simulink model "P702_NI_SoftECU"  (R2019a)
settings: Solver=ode1  StartTime=0.0  StopTime=Inf  FixedStep=0.001  RelTol=1e-3  EnableMultiTasking=on
PreLoadFcn:
  | run '.\VeriStand_BlockSet\NIVeriStandAddPaths.m'
undefined symbols (not defined in the file or in its folder): magnitude
libraries: simulink x83, simulink_extras x1
(part 43 of 76)

== system P702_NI_SoftECU/Input/GWM-SCCM//PDB//RCM//GSM/GSM/Gear_Shift_by_Wire_FD1 ==
  BrkSwtchPos_B_ActlGsm : S-Function  Priority=1  FunctionName=NIVeriStandIO  Parameters=width dtype portnum stime stype btype  SFunctionDeploymentMode=off  EnableBusSupport=off  mask(NI VeriStand Inport){portnum=1, width=-1, stime=-1, dtype=auto, stype=auto, btype=1}
      mask prompts: portnum "Port number:"; width "Port dimensions (-1 for dynamically sized):"; stime "Sample time (-1 for inherited):"; dtype "Data type:"; stype "Signal type:"; btype "Block type:"
      mask help: Use this inport on any level of nested subsystems to allow NI VeriStand software to map signals to it.
      mask init:
      | NIVeriStandIO_init;
      settings: CopyFcn=NIVeriStand_MDL_functions('', 'IO_copy');  DeleteFcn=NIVeriStand_MDL_functions('', 'IO_delete');  MoveFcn=set_param(gcb, 'Mask', 'on');
      mask Callback portnum: NIVeriStand_MDL_functions('', 'IO_setportnum');
      mask TypeOptions dtype: auto | double | single | int8 | uint8 | int16 | uint16 | int32 | uint32 | boolean
      mask Callback dtype: NIVeriStand_MDL_functions('', 'IO_booleansignal');
      mask TypeOptions stype: auto | real | complex
      mask Display:
      | patch([-x x], [-y y], [.90980 .81960 .32156]);
      | plot([xrad -x x xrad], [yrad -y y yrad]);
      | fprintf('NI In%d', portnum);
  Bus_Sig : BusCreator  Inputs=28
  DrQltyDrv_D_StatGsm : S-Function  Priority=2  FunctionName=NIVeriStandIO  Parameters=width dtype portnum stime stype btype  SFunctionDeploymentMode=off  EnableBusSupport=off  mask(NI VeriStand Inport){portnum=2, width=-1, stime=-1, dtype=auto, stype=auto, btype=1}
      mask prompts: portnum "Port number:"; width "Port dimensions (-1 for dynamically sized):"; stime "Sample time (-1 for inherited):"; dtype "Data type:"; stype "Signal type:"; btype "Block type:"
      mask help: Use this inport on any level of nested subsystems to allow NI VeriStand software to map signals to it.
      mask init:
      | NIVeriStandIO_init;
      settings: CopyFcn=NIVeriStand_MDL_functions('', 'IO_copy');  DeleteFcn=NIVeriStand_MDL_functions('', 'IO_delete');  MoveFcn=set_param(gcb, 'Mask', 'on');
      mask Callback portnum: NIVeriStand_MDL_functions('', 'IO_setportnum');
      mask TypeOptions dtype: auto | double | single | int8 | uint8 | int16 | uint16 | int32 | uint32 | boolean
      mask Callback dtype: NIVeriStand_MDL_functions('', 'IO_booleansignal');
      mask TypeOptions stype: auto | real | complex
      mask Display:
      | patch([-x x], [-y y], [.90980 .81960 .32156]);
      | plot([xrad -x x xrad], [yrad -y y yrad]);
      | fprintf('NI In%d', portnum);
  GsmGearMsgTxt_D_Rq : S-Function  Priority=3  FunctionName=NIVeriStandIO  Parameters=width dtype portnum stime stype btype  SFunctionDeploymentMode=off  EnableBusSupport=off  mask(NI VeriStand Inport){portnum=3, width=-1, stime=-1, dtype=auto, stype=auto, btype=1}
      mask prompts: portnum "Port number:"; width "Port dimensions (-1 for dynamically sized):"; stime "Sample time (-1 for inherited):"; dtype "Data type:"; stype "Signal type:"; btype "Block type:"
      mask help: Use this inport on any level of nested subsystems to allow NI VeriStand software to map signals to it.
      mask init:
      | NIVeriStandIO_init;
      settings: CopyFcn=NIVeriStand_MDL_functions('', 'IO_copy');  DeleteFcn=NIVeriStand_MDL_functions('', 'IO_delete');  MoveFcn=set_param(gcb, 'Mask', 'on');
      mask Callback portnum: NIVeriStand_MDL_functions('', 'IO_setportnum');
      mask TypeOptions dtype: auto | double | single | int8 | uint8 | int16 | uint16 | int32 | uint32 | boolean
      mask Callback dtype: NIVeriStand_MDL_functions('', 'IO_booleansignal');
      mask TypeOptions stype: auto | real | complex
      mask Display:
      | patch([-x x], [-y y], [.90980 .81960 .32156]);
      | plot([xrad -x x xrad], [yrad -y y yrad]);
      | fprintf('NI In%d', portnum);
  PrkBrkActv_D_RqGsmGear : S-Function  Priority=4  FunctionName=NIVeriStandIO  Parameters=width dtype portnum stime stype btype  SFunctionDeploymentMode=off  EnableBusSupport=off  mask(NI VeriStand Inport){portnum=4, width=-1, stime=-1, dtype=auto, stype=auto, btype=1}
      mask prompts: portnum "Port number:"; width "Port dimensions (-1 for dynamically sized):"; stime "Sample time (-1 for inherited):"; dtype "Data type:"; stype "Signal type:"; btype "Block type:"
      mask help: Use this inport on any level of nested subsystems to allow NI VeriStand software to map signals to it.
      mask init:
      | NIVeriStandIO_init;
      settings: CopyFcn=NIVeriStand_MDL_functions('', 'IO_copy');  DeleteFcn=NIVeriStand_MDL_functions('', 'IO_delete');  MoveFcn=set_param(gcb, 'Mask', 'on');
      mask Callback portnum: NIVeriStand_MDL_functions('', 'IO_setportnum');
      mask TypeOptions dtype: auto | double | single | int8 | uint8 | int16 | uint16 | int32 | uint32 | boolean
      mask Callback dtype: NIVeriStand_MDL_functions('', 'IO_booleansignal');
      mask TypeOptions stype: auto | real | complex
      mask Display:
      | patch([-x x], [-y y], [.90980 .81960 .32156]);
      | plot([xrad -x x xrad], [yrad -y y yrad]);
      | fprintf('NI In%d', portnum);
  TrnBtsiOvrrd_B_Stat : S-Function  Priority=5  FunctionName=NIVeriStandIO  Parameters=width dtype portnum stime stype btype  SFunctionDeploymentMode=off  EnableBusSupport=off  mask(NI VeriStand Inport){portnum=5, width=-1, stime=-1, dtype=auto, stype=auto, btype=1}
      mask prompts: portnum "Port number:"; width "Port dimensions (-1 for dynamically sized):"; stime "Sample time (-1 for inherited):"; dtype "Data type:"; stype "Signal type:"; btype "Block type:"
      mask help: Use this inport on any level of nested subsystems to allow NI VeriStand software to map signals to it.
      mask init:
      | NIVeriStandIO_init;
      settings: CopyFcn=NIVeriStand_MDL_functions('', 'IO_copy');  DeleteFcn=NIVeriStand_MDL_functions('', 'IO_delete');  MoveFcn=set_param(gcb, 'Mask', 'on');
      mask Callback portnum: NIVeriStand_MDL_functions('', 'IO_setportnum');
      mask TypeOptions dtype: auto | double | single | int8 | uint8 | int16 | uint16 | int32 | uint32 | boolean
      mask Callback dtype: NIVeriStand_MDL_functions('', 'IO_booleansignal');
      mask TypeOptions stype: auto | real | complex
      mask Display:
      | patch([-x x], [-y y], [.90980 .81960 .32156]);
      | plot([xrad -x x xrad], [yrad -y y yrad]);
      | fprintf('NI In%d', portnum);
  TrnGearButtn_B_ActlD0 : S-Function  Priority=6  FunctionName=NIVeriStandIO  Parameters=width dtype portnum stime stype btype  SFunctionDeploymentMode=off  EnableBusSupport=off  mask(NI VeriStand Inport){portnum=6, width=-1, stime=-1, dtype=auto, stype=auto, btype=1}
      mask prompts: portnum "Port number:"; width "Port dimensions (-1 for dynamically sized):"; stime "Sample time (-1 for inherited):"; dtype "Data type:"; stype "Signal type:"; btype "Block type:"
      mask help: Use this inport on any level of nested subsystems to allow NI VeriStand software to map signals to it.
      mask init:
      | NIVeriStandIO_init;
      settings: CopyFcn=NIVeriStand_MDL_functions('', 'IO_copy');  DeleteFcn=NIVeriStand_MDL_functions('', 'IO_delete');  MoveFcn=set_param(gcb, 'Mask', 'on');
      mask Callback portnum: NIVeriStand_MDL_functions('', 'IO_setportnum');
      mask TypeOptions dtype: auto | double | single | int8 | uint8 | int16 | uint16 | int32 | uint32 | boolean
      mask Callback dtype: NIVeriStand_MDL_functions('', 'IO_booleansignal');
      mask TypeOptions stype: auto | real | complex
      mask Display:
      | patch([-x x], [-y y], [.90980 .81960 .32156]);
      | plot([xrad -x x xrad], [yrad -y y yrad]);
      | fprintf('NI In%d', portnum);
  TrnGearButtn_B_ActlD1 : S-Function  Priority=7  FunctionName=NIVeriStandIO  Parameters=width dtype portnum stime stype btype  SFunctionDeploymentMode=off  EnableBusSupport=off  mask(NI VeriStand Inport){portnum=7, width=-1, stime=-1, dtype=auto, stype=auto, btype=1}
      mask prompts: portnum "Port number:"; width "Port dimensions (-1 for dynamically sized):"; stime "Sample time (-1 for inherited):"; dtype "Data type:"; stype "Signal type:"; btype "Block type:"
      mask help: Use this inport on any level of nested subsystems to allow NI VeriStand software to map signals to it.
      mask init:
      | NIVeriStandIO_init;
      settings: CopyFcn=NIVeriStand_MDL_functions('', 'IO_copy');  DeleteFcn=NIVeriStand_MDL_functions('', 'IO_delete');  MoveFcn=set_param(gcb, 'Mask', 'on');
      mask Callback portnum: NIVeriStand_MDL_functions('', 'IO_setportnum');
      mask TypeOptions dtype: auto | double | single | int8 | uint8 | int16 | uint16 | int32 | uint32 | boolean
      mask Callback dtype: NIVeriStand_MDL_functions('', 'IO_booleansignal');
      mask TypeOptions stype: auto | real | complex
      mask Display:
      | patch([-x x], [-y y], [.90980 .81960 .32156]);
      | plot([xrad -x x xrad], [yrad -y y yrad]);
      | fprintf('NI In%d', portnum);
  TrnGearButtn_B_ActlD2 : S-Function  Priority=8  FunctionName=NIVeriStandIO  Parameters=width dtype portnum stime stype btype  SFunctionDeploymentMode=off  EnableBusSupport=off  mask(NI VeriStand Inport){portnum=8, width=-1, stime=-1, dtype=auto, stype=auto, btype=1}
      mask prompts: portnum "Port number:"; width "Port dimensions (-1 for dynamically sized):"; stime "Sample time (-1 for inherited):"; dtype "Data type:"; stype "Signal type:"; btype "Block type:"
      mask help: Use this inport on any level of nested subsystems to allow NI VeriStand software to map signals to it.
      mask init:
      | NIVeriStandIO_init;
      settings: CopyFcn=NIVeriStand_MDL_functions('', 'IO_copy');  DeleteFcn=NIVeriStand_MDL_functions('', 'IO_delete');  MoveFcn=set_param(gcb, 'Mask', 'on');
      mask Callback portnum: NIVeriStand_MDL_functions('', 'IO_setportnum');
      mask TypeOptions dtype: auto | double | single | int8 | uint8 | int16 | uint16 | int32 | uint32 | boolean
      mask Callback dtype: NIVeriStand_MDL_functions('', 'IO_booleansignal');
      mask TypeOptions stype: auto | real | complex
      mask Display:
      | patch([-x x], [-y y], [.90980 .81960 .32156]);
      | plot([xrad -x x xrad], [yrad -y y yrad]);
      | fprintf('NI In%d', portnum);
  TrnGearButtn_B_ActlM0 : S-Function  Priority=9  FunctionName=NIVeriStandIO  Parameters=width dtype portnum stime stype btype  SFunctionDeploymentMode=off  EnableBusSupport=off  mask(NI VeriStand Inport){portnum=9, width=-1, stime=-1, dtype=auto, stype=auto, btype=1}
      mask prompts: portnum "Port number:"; width "Port dimensions (-1 for dynamically sized):"; stime "Sample time (-1 for inherited):"; dtype "Data type:"; stype "Signal type:"; btype "Block type:"
      mask help: Use this inport on any level of nested subsystems to allow NI VeriStand software to map signals to it.
      mask init:
      | NIVeriStandIO_init;
      settings: CopyFcn=NIVeriStand_MDL_functions('', 'IO_copy');  DeleteFcn=NIVeriStand_MDL_functions('', 'IO_delete');  MoveFcn=set_param(gcb, 'Mask', 'on');
      mask Callback portnum: NIVeriStand_MDL_functions('', 'IO_setportnum');
      mask TypeOptions dtype: auto | double | single | int8 | uint8 | int16 | uint16 | int32 | uint32 | boolean
      mask Callback dtype: NIVeriStand_MDL_functions('', 'IO_booleansignal');
      mask TypeOptions stype: auto | real | complex
      mask Display:
      | patch([-x x], [-y y], [.90980 .81960 .32156]);
      | plot([xrad -x x xrad], [yrad -y y yrad]);
      | fprintf('NI In%d', portnum);
  TrnGearButtn_B_ActlM1 : S-Function  Priority=10  FunctionName=NIVeriStandIO  Parameters=width dtype portnum stime stype btype  SFunctionDeploymentMode=off  EnableBusSupport=off  mask(NI VeriStand Inport){portnum=10, width=-1, stime=-1, dtype=auto, stype=auto, btype=1}
      mask prompts: portnum "Port number:"; width "Port dimensions (-1 for dynamically sized):"; stime "Sample time (-1 for inherited):"; dtype "Data type:"; stype "Signal type:"; btype "Block type:"
      mask help: Use this inport on any level of nested subsystems to allow NI VeriStand software to map signals to it.
      mask init:
      | NIVeriStandIO_init;
      settings: CopyFcn=NIVeriStand_MDL_functions('', 'IO_copy');  DeleteFcn=NIVeriStand_MDL_functions('', 'IO_delete');  MoveFcn=set_param(gcb, 'Mask', 'on');
      mask Callback portnum: NIVeriStand_MDL_functions('', 'IO_setportnum');
      mask TypeOptions dtype: auto | double | single | int8 | uint8 | int16 | uint16 | int32 | uint32 | boolean
      mask Callback dtype: NIVeriStand_MDL_functions('', 'IO_booleansignal');
      mask TypeOptions stype: auto | real | complex
      mask Display:
      | patch([-x x], [-y y], [.90980 .81960 .32156]);
      | plot([xrad -x x xrad], [yrad -y y yrad]);
      | fprintf('NI In%d', portnum);
  TrnGearButtn_B_ActlM2 : S-Function  Priority=11  FunctionName=NIVeriStandIO  Parameters=width dtype portnum stime stype btype  SFunctionDeploymentMode=off  EnableBusSupport=off  mask(NI VeriStand Inport){portnum=11, width=-1, stime=-1, dtype=auto, stype=auto, btype=1}
      mask prompts: portnum "Port number:"; width "Port dimensions (-1 for dynamically sized):"; stime "Sample time (-1 for inherited):"; dtype "Data type:"; stype "Signal type:"; btype "Block type:"
      mask help: Use this inport on any level of nested subsystems to allow NI VeriStand software to map signals to it.
      mask init:
      | NIVeriStandIO_init;
      settings: CopyFcn=NIVeriStand_MDL_functions('', 'IO_copy');  DeleteFcn=NIVeriStand_MDL_functions('', 'IO_delete');  MoveFcn=set_param(gcb, 'Mask', 'on');
      mask Callback portnum: NIVeriStand_MDL_functions('', 'IO_setportnum');
      mask TypeOptions dtype: auto | double | single | int8 | uint8 | int16 | uint16 | int32 | uint32 | boolean
      mask Callback dtype: NIVeriStand_MDL_functions('', 'IO_booleansignal');
      mask TypeOptions stype: auto | real | complex
      mask Display:
      | patch([-x x], [-y y], [.90980 .81960 .32156]);
      | plot([xrad -x x xrad], [yrad -y y yrad]);
      | fprintf('NI In%d', portnum);
  TrnGearButtn_B_ActlN0 : S-Function  Priority=12  FunctionName=NIVeriStandIO  Parameters=width dtype portnum stime stype btype  SFunctionDeploymentMode=off  EnableBusSupport=off  mask(NI VeriStand Inport){portnum=12, width=-1, stime=-1, dtype=auto, stype=auto, btype=1}
      mask prompts: portnum "Port number:"; width "Port dimensions (-1 for dynamically sized):"; stime "Sample time (-1 for inherited):"; dtype "Data type:"; stype "Signal type:"; btype "Block type:"
      mask help: Use this inport on any level of nested subsystems to allow NI VeriStand software to map signals to it.
      mask init:
      | NIVeriStandIO_init;
      settings: CopyFcn=NIVeriStand_MDL_functions('', 'IO_copy');  DeleteFcn=NIVeriStand_MDL_functions('', 'IO_delete');  MoveFcn=set_param(gcb, 'Mask', 'on');
      mask Callback portnum: NIVeriStand_MDL_functions('', 'IO_setportnum');
      mask TypeOptions dtype: auto | double | single | int8 | uint8 | int16 | uint16 | int32 | uint32 | boolean
      mask Callback dtype: NIVeriStand_MDL_functions('', 'IO_booleansignal');
      mask TypeOptions stype: auto | real | complex
      mask Display:
      | patch([-x x], [-y y], [.90980 .81960 .32156]);
      | plot([xrad -x x xrad], [yrad -y y yrad]);
      | fprintf('NI In%d', portnum);
  TrnGearButtn_B_ActlN1 : S-Function  Priority=13  FunctionName=NIVeriStandIO  Parameters=width dtype portnum stime stype btype  SFunctionDeploymentMode=off  EnableBusSupport=off  mask(NI VeriStand Inport){portnum=13, width=-1, stime=-1, dtype=auto, stype=auto, btype=1}
      mask prompts: portnum "Port number:"; width "Port dimensions (-1 for dynamically sized):"; stime "Sample time (-1 for inherited):"; dtype "Data type:"; stype "Signal type:"; btype "Block type:"
      mask help: Use this inport on any level of nested subsystems to allow NI VeriStand software to map signals to it.
      mask init:
      | NIVeriStandIO_init;
      settings: CopyFcn=NIVeriStand_MDL_functions('', 'IO_copy');  DeleteFcn=NIVeriStand_MDL_functions('', 'IO_delete');  MoveFcn=set_param(gcb, 'Mask', 'on');
      mask Callback portnum: NIVeriStand_MDL_functions('', 'IO_setportnum');
      mask TypeOptions dtype: auto | double | single | int8 | uint8 | int16 | uint16 | int32 | uint32 | boolean
      mask Callback dtype: NIVeriStand_MDL_functions('', 'IO_booleansignal');
      mask TypeOptions stype: auto | real | complex
      mask Display:
      | patch([-x x], [-y y], [.90980 .81960 .32156]);
      | plot([xrad -x x xrad], [yrad -y y yrad]);
      | fprintf('NI In%d', portnum);
  TrnGearButtn_B_ActlN2 : S-Function  Priority=14  FunctionName=NIVeriStandIO  Parameters=width dtype portnum stime stype btype  SFunctionDeploymentMode=off  EnableBusSupport=off  mask(NI VeriStand Inport){portnum=14, width=-1, stime=-1, dtype=auto, stype=auto, btype=1}
      mask prompts: portnum "Port number:"; width "Port dimensions (-1 for dynamically sized):"; stime "Sample time (-1 for inherited):"; dtype "Data type:"; stype "Signal type:"; btype "Block type:"
      mask help: Use this inport on any level of nested subsystems to allow NI VeriStand software to map signals to it.
      mask init:
      | NIVeriStandIO_init;
      settings: CopyFcn=NIVeriStand_MDL_functions('', 'IO_copy');  DeleteFcn=NIVeriStand_MDL_functions('', 'IO_delete');  MoveFcn=set_param(gcb, 'Mask', 'on');
      mask Callback portnum: NIVeriStand_MDL_functions('', 'IO_setportnum');
      mask TypeOptions dtype: auto | double | single | int8 | uint8 | int16 | uint16 | int32 | uint32 | boolean
      mask Callback dtype: NIVeriStand_MDL_functions('', 'IO_booleansignal');
      mask TypeOptions stype: auto | real | complex
      mask Display:
      | patch([-x x], [-y y], [.90980 .81960 .32156]);
      | plot([xrad -x x xrad], [yrad -y y yrad]);
      | fprintf('NI In%d', portnum);
  TrnGearButtn_B_ActlP0 : S-Function  Priority=15  FunctionName=NIVeriStandIO  Parameters=width dtype portnum stime stype btype  SFunctionDeploymentMode=off  EnableBusSupport=off  mask(NI VeriStand Inport){portnum=15, width=-1, stime=-1, dtype=auto, stype=auto, btype=1}
      mask prompts: portnum "Port number:"; width "Port dimensions (-1 for dynamically sized):"; stime "Sample time (-1 for inherited):"; dtype "Data type:"; stype "Signal type:"; btype "Block type:"
      mask help: Use this inport on any level of nested subsystems to allow NI VeriStand software to map signals to it.
      mask init:
      | NIVeriStandIO_init;
      settings: CopyFcn=NIVeriStand_MDL_functions('', 'IO_copy');  DeleteFcn=NIVeriStand_MDL_functions('', 'IO_delete');  MoveFcn=set_param(gcb, 'Mask', 'on');
      mask Callback portnum: NIVeriStand_MDL_functions('', 'IO_setportnum');
      mask TypeOptions dtype: auto | double | single | int8 | uint8 | int16 | uint16 | int32 | uint32 | boolean
      mask Callback dtype: NIVeriStand_MDL_functions('', 'IO_booleansignal');
      mask TypeOptions stype: auto | real | complex
      mask Display:
      | patch([-x x], [-y y], [.90980 .81960 .32156]);
      | plot([xrad -x x xrad], [yrad -y y yrad]);
      | fprintf('NI In%d', portnum);
  TrnGearButtn_B_ActlP1 : S-Function  Priority=16  FunctionName=NIVeriStandIO  Parameters=width dtype portnum stime stype btype  SFunctionDeploymentMode=off  EnableBusSupport=off  mask(NI VeriStand Inport){portnum=16, width=-1, stime=-1, dtype=auto, stype=auto, btype=1}
      mask prompts: portnum "Port number:"; width "Port dimensions (-1 for dynamically sized):"; stime "Sample time (-1 for inherited):"; dtype "Data type:"; stype "Signal type:"; btype "Block type:"
      mask help: Use this inport on any level of nested subsystems to allow NI VeriStand software to map signals to it.
      mask init:
      | NIVeriStandIO_init;
      settings: CopyFcn=NIVeriStand_MDL_functions('', 'IO_copy');  DeleteFcn=NIVeriStand_MDL_functions('', 'IO_delete');  MoveFcn=set_param(gcb, 'Mask', 'on');
      mask Callback portnum: NIVeriStand_MDL_functions('', 'IO_setportnum');
      mask TypeOptions dtype: auto | double | single | int8 | uint8 | int16 | uint16 | int32 | uint32 | boolean
      mask Callback dtype: NIVeriStand_MDL_functions('', 'IO_booleansignal');
      mask TypeOptions stype: auto | real | complex
      mask Display:
      | patch([-x x], [-y y], [.90980 .81960 .32156]);
      | plot([xrad -x x xrad], [yrad -y y yrad]);
      | fprintf('NI In%d', portnum);
  TrnGearButtn_B_ActlP2 : S-Function  Priority=17  FunctionName=NIVeriStandIO  Parameters=width dtype portnum stime stype btype  SFunctionDeploymentMode=off  EnableBusSupport=off  mask(NI VeriStand Inport){portnum=17, width=-1, stime=-1, dtype=auto, stype=auto, btype=1}
      mask prompts: portnum "Port number:"; width "Port dimensions (-1 for dynamically sized):"; stime "Sample time (-1 for inherited):"; dtype "Data type:"; stype "Signal type:"; btype "Block type:"
      mask help: Use this inport on any level of nested subsystems to allow NI VeriStand software to map signals to it.
      mask init:
      | NIVeriStandIO_init;
      settings: CopyFcn=NIVeriStand_MDL_functions('', 'IO_copy');  DeleteFcn=NIVeriStand_MDL_functions('', 'IO_delete');  MoveFcn=set_param(gcb, 'Mask', 'on');
      mask Callback portnum: NIVeriStand_MDL_functions('', 'IO_setportnum');
      mask TypeOptions dtype: auto | double | single | int8 | uint8 | int16 | uint16 | int32 | uint32 | boolean
      mask Callback dtype: NIVeriStand_MDL_functions('', 'IO_booleansignal');
      mask TypeOptions stype: auto | real | complex
      mask Display:
      | patch([-x x], [-y y], [.90980 .81960 .32156]);
      | plot([xrad -x x xrad], [yrad -y y yrad]);
      | fprintf('NI In%d', portnum);
  TrnGearButtn_B_ActlR0 : S-Function  Priority=18  FunctionName=NIVeriStandIO  Parameters=width dtype portnum stime stype btype  SFunctionDeploymentMode=off  EnableBusSupport=off  mask(NI VeriStand Inport){portnum=18, width=-1, stime=-1, dtype=auto, stype=auto, btype=1}
      mask prompts: portnum "Port number:"; width "Port dimensions (-1 for dynamically sized):"; stime "Sample time (-1 for inherited):"; dtype "Data type:"; stype "Signal type:"; btype "Block type:"
      mask help: Use this inport on any level of nested subsystems to allow NI VeriStand software to map signals to it.
      mask init:
      | NIVeriStandIO_init;
      settings: CopyFcn=NIVeriStand_MDL_functions('', 'IO_copy');  DeleteFcn=NIVeriStand_MDL_functions('', 'IO_delete');  MoveFcn=set_param(gcb, 'Mask', 'on');
      mask Callback portnum: NIVeriStand_MDL_functions('', 'IO_setportnum');
      mask TypeOptions dtype: auto | double | single | int8 | uint8 | int16 | uint16 | int32 | uint32 | boolean
      mask Callback dtype: NIVeriStand_MDL_functions('', 'IO_booleansignal');
      mask TypeOptions stype: auto | real | complex
      mask Display:
      | patch([-x x], [-y y], [.90980 .81960 .32156]);
      | plot([xrad -x x xrad], [yrad -y y yrad]);
      | fprintf('NI In%d', portnum);
  TrnGearButtn_B_ActlR1 : S-Function  Priority=19  FunctionName=NIVeriStandIO  Parameters=width dtype portnum stime stype btype  SFunctionDeploymentMode=off  EnableBusSupport=off  mask(NI VeriStand Inport){portnum=19, width=-1, stime=-1, dtype=auto, stype=auto, btype=1}
      mask prompts: portnum "Port number:"; width "Port dimensions (-1 for dynamically sized):"; stime "Sample time (-1 for inherited):"; dtype "Data type:"; stype "Signal type:"; btype "Block type:"
      mask help: Use this inport on any level of nested subsystems to allow NI VeriStand software to map signals to it.
      mask init:
      | NIVeriStandIO_init;
      settings: CopyFcn=NIVeriStand_MDL_functions('', 'IO_copy');  DeleteFcn=NIVeriStand_MDL_functions('', 'IO_delete');  MoveFcn=set_param(gcb, 'Mask', 'on');
      mask Callback portnum: NIVeriStand_MDL_functions('', 'IO_setportnum');
      mask TypeOptions dtype: auto | double | single | int8 | uint8 | int16 | uint16 | int32 | uint32 | boolean
      mask Callback dtype: NIVeriStand_MDL_functions('', 'IO_booleansignal');
      mask TypeOptions stype: auto | real | complex
      mask Display:
      | patch([-x x], [-y y], [.90980 .81960 .32156]);
      | plot([xrad -x x xrad], [yrad -y y yrad]);
      | fprintf('NI In%d', portnum);
  TrnGearButtn_B_ActlR2 : S-Function  Priority=20  FunctionName=NIVeriStandIO  Parameters=width dtype portnum stime stype btype  SFunctionDeploymentMode=off  EnableBusSupport=off  mask(NI VeriStand Inport){portnum=20, width=-1, stime=-1, dtype=auto, stype=auto, btype=1}
      mask prompts: portnum "Port number:"; width "Port dimensions (-1 for dynamically sized):"; stime "Sample time (-1 for inherited):"; dtype "Data type:"; stype "Signal type:"; btype "Block type:"
      mask help: Use this inport on any level of nested subsystems to allow NI VeriStand software to map signals to it.
      mask init:
      | NIVeriStandIO_init;
      settings: CopyFcn=NIVeriStand_MDL_functions('', 'IO_copy');  DeleteFcn=NIVeriStand_MDL_functions('', 'IO_delete');  MoveFcn=set_param(gcb, 'Mask', 'on');
      mask Callback portnum: NIVeriStand_MDL_functions('', 'IO_setportnum');
      mask TypeOptions dtype: auto | double | single | int8 | uint8 | int16 | uint16 | int32 | uint32 | boolean
      mask Callback dtype: NIVeriStand_MDL_functions('', 'IO_booleansignal');
      mask TypeOptions stype: auto | real | complex
      mask Display:
      | patch([-x x], [-y y], [.90980 .81960 .32156]);
      | plot([xrad -x x xrad], [yrad -y y yrad]);
      | fprintf('NI In%d', portnum);
  TrnGearButtn_U_Actl : S-Function  Priority=21  FunctionName=NIVeriStandIO  Parameters=width dtype portnum stime stype btype  SFunctionDeploymentMode=off  EnableBusSupport=off  mask(NI VeriStand Inport){portnum=21, width=-1, stime=-1, dtype=auto, stype=auto, btype=1}
      mask prompts: portnum "Port number:"; width "Port dimensions (-1 for dynamically sized):"; stime "Sample time (-1 for inherited):"; dtype "Data type:"; stype "Signal type:"; btype "Block type:"
      mask help: Use this inport on any level of nested subsystems to allow NI VeriStand software to map signals to it.
      mask init:
      | NIVeriStandIO_init;
      settings: CopyFcn=NIVeriStand_MDL_functions('', 'IO_copy');  DeleteFcn=NIVeriStand_MDL_functions('', 'IO_delete');  MoveFcn=set_param(gcb, 'Mask', 'on');
      mask Callback portnum: NIVeriStand_MDL_functions('', 'IO_setportnum');
      mask TypeOptions dtype: auto | double | single | int8 | uint8 | int16 | uint16 | int32 | uint32 | boolean
      mask Callback dtype: NIVeriStand_MDL_functions('', 'IO_booleansignal');
      mask TypeOptions stype: auto | real | complex
      mask Display:
      | patch([-x x], [-y y], [.90980 .81960 .32156]);
      | plot([xrad -x x xrad], [yrad -y y yrad]);
      | fprintf('NI In%d', portnum);
  TrnGearRqCnt_B_Actl : S-Function  Priority=22  FunctionName=NIVeriStandIO  Parameters=width dtype portnum stime stype btype  SFunctionDeploymentMode=off  EnableBusSupport=off  mask(NI VeriStand Inport){portnum=22, width=-1, stime=-1, dtype=auto, stype=auto, btype=1}
      mask prompts: portnum "Port number:"; width "Port dimensions (-1 for dynamically sized):"; stime "Sample time (-1 for inherited):"; dtype "Data type:"; stype "Signal type:"; btype "Block type:"
      mask help: Use this inport on any level of nested subsystems to allow NI VeriStand software to map signals to it.
      mask init:
      | NIVeriStandIO_init;
      settings: CopyFcn=NIVeriStand_MDL_functions('', 'IO_copy');  DeleteFcn=NIVeriStand_MDL_functions('', 'IO_delete');  MoveFcn=set_param(gcb, 'Mask', 'on');
      mask Callback portnum: NIVeriStand_MDL_functions('', 'IO_setportnum');
      mask TypeOptions dtype: auto | double | single | int8 | uint8 | int16 | uint16 | int32 | uint32 | boolean
      mask Callback dtype: NIVeriStand_MDL_functions('', 'IO_booleansignal');
      mask TypeOptions stype: auto | real | complex
      mask Display:
      | patch([-x x], [-y y], [.90980 .81960 .32156]);
      | plot([xrad -x x xrad], [yrad -y y yrad]);
      | fprintf('NI In%d', portnum);
  TrnGear_D_RqDrv : S-Function  Priority=23  FunctionName=NIVeriStandIO  Parameters=width dtype portnum stime stype btype  SFunctionDeploymentMode=off  EnableBusSupport=off  mask(NI VeriStand Inport){portnum=23, width=-1, stime=-1, dtype=auto, stype=auto, btype=1}
      mask prompts: portnum "Port number:"; width "Port dimensions (-1 for dynamically sized):"; stime "Sample time (-1 for inherited):"; dtype "Data type:"; stype "Signal type:"; btype "Block type:"
      mask help: Use this inport on any level of nested subsystems to allow NI VeriStand software to map signals to it.
      mask init:
      | NIVeriStandIO_init;
      settings: CopyFcn=NIVeriStand_MDL_functions('', 'IO_copy');  DeleteFcn=NIVeriStand_MDL_functions('', 'IO_delete');  MoveFcn=set_param(gcb, 'Mask', 'on');
      mask Callback portnum: NIVeriStand_MDL_functions('', 'IO_setportnum');
      mask TypeOptions dtype: auto | double | single | int8 | uint8 | int16 | uint16 | int32 | uint32 | boolean
      mask Callback dtype: NIVeriStand_MDL_functions('', 'IO_booleansignal');
      mask TypeOptions stype: auto | real | complex
      mask Display:
      | patch([-x x], [-y y], [.90980 .81960 .32156]);
      | plot([xrad -x x xrad], [yrad -y y yrad]);
      | fprintf('NI In%d', portnum);
  TrnGear_No_Cnt : S-Function  Priority=24  FunctionName=NIVeriStandIO  Parameters=width dtype portnum stime stype btype  SFunctionDeploymentMode=off  EnableBusSupport=off  mask(NI VeriStand Inport){portnum=24, width=-1, stime=-1, dtype=auto, stype=auto, btype=1}
      mask prompts: portnum "Port number:"; width "Port dimensions (-1 for dynamically sized):"; stime "Sample time (-1 for inherited):"; dtype "Data type:"; stype "Signal type:"; btype "Block type:"
      mask help: Use this inport on any level of nested subsystems to allow NI VeriStand software to map signals to it.
      mask init:
      | NIVeriStandIO_init;
      settings: CopyFcn=NIVeriStand_MDL_functions('', 'IO_copy');  DeleteFcn=NIVeriStand_MDL_functions('', 'IO_delete');  MoveFcn=set_param(gcb, 'Mask', 'on');
      mask Callback portnum: NIVeriStand_MDL_functions('', 'IO_setportnum');
      mask TypeOptions dtype: auto | double | single | int8 | uint8 | int16 | uint16 | int32 | uint32 | boolean
      mask Callback dtype: NIVeriStand_MDL_functions('', 'IO_booleansignal');
      mask TypeOptions stype: auto | real | complex
      mask Display:
      | patch([-x x], [-y y], [.90980 .81960 .32156]);
      | plot([xrad -x x xrad], [yrad -y y yrad]);
      | fprintf('NI In%d', portnum);
  TrnGear_No_Cs : S-Function  Priority=25  FunctionName=NIVeriStandIO  Parameters=width dtype portnum stime stype btype  SFunctionDeploymentMode=off  EnableBusSupport=off  mask(NI VeriStand Inport){portnum=25, width=-1, stime=-1, dtype=auto, stype=auto, btype=1}
      mask prompts: portnum "Port number:"; width "Port dimensions (-1 for dynamically sized):"; stime "Sample time (-1 for inherited):"; dtype "Data type:"; stype "Signal type:"; btype "Block type:"
      mask help: Use this inport on any level of nested subsystems to allow NI VeriStand software to map signals to it.
      mask init:
      | NIVeriStandIO_init;
      settings: CopyFcn=NIVeriStand_MDL_functions('', 'IO_copy');  DeleteFcn=NIVeriStand_MDL_functions('', 'IO_delete');  MoveFcn=set_param(gcb, 'Mask', 'on');
      mask Callback portnum: NIVeriStand_MDL_functions('', 'IO_setportnum');
      mask TypeOptions dtype: auto | double | single | int8 | uint8 | int16 | uint16 | int32 | uint32 | boolean
      mask Callback dtype: NIVeriStand_MDL_functions('', 'IO_booleansignal');
      mask TypeOptions stype: auto | real | complex
      mask Display:
      | patch([-x x], [-y y], [.90980 .81960 .32156]);
      | plot([xrad -x x xrad], [yrad -y y yrad]);
      | fprintf('NI In%d', portnum);
  TrnGsmNtmState_D_Actl : S-Function  Priority=26  FunctionName=NIVeriStandIO  Parameters=width dtype portnum stime stype btype  SFunctionDeploymentMode=off  EnableBusSupport=off  mask(NI VeriStand Inport){portnum=26, width=-1, stime=-1, dtype=auto, stype=auto, btype=1}
      mask prompts: portnum "Port number:"; width "Port dimensions (-1 for dynamically sized):"; stime "Sample time (-1 for inherited):"; dtype "Data type:"; stype "Signal type:"; btype "Block type:"
      mask help: Use this inport on any level of nested subsystems to allow NI VeriStand software to map signals to it.
      mask init:
      | NIVeriStandIO_init;
      settings: CopyFcn=NIVeriStand_MDL_functions('', 'IO_copy');  DeleteFcn=NIVeriStand_MDL_functions('', 'IO_delete');  MoveFcn=set_param(gcb, 'Mask', 'on');
      mask Callback portnum: NIVeriStand_MDL_functions('', 'IO_setportnum');
      mask TypeOptions dtype: auto | double | single | int8 | uint8 | int16 | uint16 | int32 | uint32 | boolean
      mask Callback dtype: NIVeriStand_MDL_functions('', 'IO_booleansignal');
      mask TypeOptions stype: auto | real | complex
      mask Display:
      | patch([-x x], [-y y], [.90980 .81960 .32156]);
      | plot([xrad -x x xrad], [yrad -y y yrad]);
      | fprintf('NI In%d', portnum);
  TrnRng_D_RqGsm : S-Function  Priority=27  FunctionName=NIVeriStandIO  Parameters=width dtype portnum stime stype btype  SFunctionDeploymentMode=off  EnableBusSupport=off  mask(NI VeriStand Inport){portnum=27, width=-1, stime=-1, dtype=auto, stype=auto, btype=1}
      mask prompts: portnum "Port number:"; width "Port dimensions (-1 for dynamically sized):"; stime "Sample time (-1 for inherited):"; dtype "Data type:"; stype "Signal type:"; btype "Block type:"
      mask help: Use this inport on any level of nested subsystems to allow NI VeriStand software to map signals to it.
      mask init:
      | NIVeriStandIO_init;
      settings: CopyFcn=NIVeriStand_MDL_functions('', 'IO_copy');  DeleteFcn=NIVeriStand_MDL_functions('', 'IO_delete');  MoveFcn=set_param(gcb, 'Mask', 'on');
      mask Callback portnum: NIVeriStand_MDL_functions('', 'IO_setportnum');
      mask TypeOptions dtype: auto | double | single | int8 | uint8 | int16 | uint16 | int32 | uint32 | boolean
      mask Callback dtype: NIVeriStand_MDL_functions('', 'IO_booleansignal');
      mask TypeOptions stype: auto | real | complex
      mask Display:
      | patch([-x x], [-y y], [.90980 .81960 .32156]);
      | plot([xrad -x x xrad], [yrad -y y yrad]);
      | fprintf('NI In%d', portnum);
  TrnValidGearRq_D_Stat : S-Function  Priority=28  FunctionName=NIVeriStandIO  Parameters=width dtype portnum stime stype btype  SFunctionDeploymentMode=off  EnableBusSupport=off  mask(NI VeriStand Inport){portnum=28, width=-1, stime=-1, dtype=auto, stype=auto, btype=1}
      mask prompts: portnum "Port number:"; width "Port dimensions (-1 for dynamically sized):"; stime "Sample time (-1 for inherited):"; dtype "Data type:"; stype "Signal type:"; btype "Block type:"
      mask help: Use this inport on any level of nested subsystems to allow NI VeriStand software to map signals to it.
      mask init:
      | NIVeriStandIO_init;
      settings: CopyFcn=NIVeriStand_MDL_functions('', 'IO_copy');  DeleteFcn=NIVeriStand_MDL_functions('', 'IO_delete');  MoveFcn=set_param(gcb, 'Mask', 'on');
      mask Callback portnum: NIVeriStand_MDL_functions('', 'IO_setportnum');
      mask TypeOptions dtype: auto | double | single | int8 | uint8 | int16 | uint16 | int32 | uint32 | boolean
      mask Callback dtype: NIVeriStand_MDL_functions('', 'IO_booleansignal');
      mask TypeOptions stype: auto | real | complex
      mask Display:
      | patch([-x x], [-y y], [.90980 .81960 .32156]);
      | plot([xrad -x x xrad], [yrad -y y yrad]);
      | fprintf('NI In%d', portnum);
  Gear_Shift_by_Wire_FD1_5A : Outport
  wires:
  Bus_Sig/1 -> Gear_Shift_by_Wire_FD1_5A/1  "Gear_Shift_by_Wire_FD1_5A"
  BrkSwtchPos_B_ActlGsm/1 -> Bus_Sig/1  "BrkSwtchPos_B_ActlGsm"
  DrQltyDrv_D_StatGsm/1 -> Bus_Sig/2  "DrQltyDrv_D_StatGsm"
  GsmGearMsgTxt_D_Rq/1 -> Bus_Sig/3  "GsmGearMsgTxt_D_Rq"
  PrkBrkActv_D_RqGsmGear/1 -> Bus_Sig/4  "PrkBrkActv_D_RqGsmGear"
  TrnBtsiOvrrd_B_Stat/1 -> Bus_Sig/5  "TrnBtsiOvrrd_B_Stat"
  TrnGearButtn_B_ActlD0/1 -> Bus_Sig/6  "TrnGearButtn_B_ActlD0"
  TrnGearButtn_B_ActlD1/1 -> Bus_Sig/7  "TrnGearButtn_B_ActlD1"
  TrnGearButtn_B_ActlD2/1 -> Bus_Sig/8  "TrnGearButtn_B_ActlD2"
  TrnGearButtn_B_ActlM0/1 -> Bus_Sig/9  "TrnGearButtn_B_ActlM0"
  TrnGearButtn_B_ActlM1/1 -> Bus_Sig/10  "TrnGearButtn_B_ActlM1"
  TrnGearButtn_B_ActlM2/1 -> Bus_Sig/11  "TrnGearButtn_B_ActlM2"
  TrnGearButtn_B_ActlN0/1 -> Bus_Sig/12  "TrnGearButtn_B_ActlN0"
  TrnGearButtn_B_ActlN1/1 -> Bus_Sig/13  "TrnGearButtn_B_ActlN1"
  TrnGearButtn_B_ActlN2/1 -> Bus_Sig/14  "TrnGearButtn_B_ActlN2"
  TrnGearButtn_B_ActlP0/1 -> Bus_Sig/15  "TrnGearButtn_B_ActlP0"
  TrnGearButtn_B_ActlP1/1 -> Bus_Sig/16  "TrnGearButtn_B_ActlP1"
  TrnGearButtn_B_ActlP2/1 -> Bus_Sig/17  "TrnGearButtn_B_ActlP2"
  TrnGearButtn_B_ActlR0/1 -> Bus_Sig/18  "TrnGearButtn_B_ActlR0"
  TrnGearButtn_B_ActlR1/1 -> Bus_Sig/19  "TrnGearButtn_B_ActlR1"
  TrnGearButtn_B_ActlR2/1 -> Bus_Sig/20  "TrnGearButtn_B_ActlR2"
  TrnGearButtn_U_Actl/1 -> Bus_Sig/21  "TrnGearButtn_U_Actl"
  TrnGearRqCnt_B_Actl/1 -> Bus_Sig/22  "TrnGearRqCnt_B_Actl"
  TrnGear_D_RqDrv/1 -> Bus_Sig/23  "TrnGear_D_RqDrv"
  TrnGear_No_Cnt/1 -> Bus_Sig/24  "TrnGear_No_Cnt"
  TrnGear_No_Cs/1 -> Bus_Sig/25  "TrnGear_No_Cs"
  TrnGsmNtmState_D_Actl/1 -> Bus_Sig/26  "TrnGsmNtmState_D_Actl"
  TrnRng_D_RqGsm/1 -> Bus_Sig/27  "TrnRng_D_RqGsm"
  TrnValidGearRq_D_Stat/1 -> Bus_Sig/28  "TrnValidGearRq_D_Stat"

== system P702_NI_SoftECU/Input/GWM-SCCM//PDB//RCM//GSM/Other_GWMTx/AC_Compressor_Data_FD1 ==
  Bus_Sig : BusCreator  Inputs=14
  ElCmprBattSysU_D_Falt : Constant  Value=0
  ElCmprBattURng_D_Falt : Constant  Value=0
  ElCmprInnrErr_D_Falt : Constant  Value=0
  ElCmprLostComm_D_Falt : Constant  Value=0
  ElCmprOverLoad_D_Falt : Constant  Value=0
  ElCmprOverTe_D_Falt : Constant  Value=0
  ElCmprOverTe_D_Stat : Constant  Value=0
  ElCmprPerfErr_D_Falt : Constant  Value=0
  ElCmprSysU_D_Falt : Constant  Value=0
  ElCmprUHi_D_Stat : Constant  Value=0
  ElCmprUHi_U_Actl : Constant  Value=0
  ElCmpr_D_Stat : Constant  Value=0
  ElCmpr_N_Actl : Constant  Value=0
  ElCmpr_Pw_Actl : Constant  Value=0
  AC_Compressor_Data_FD1_411 : Outport
  wires:
  Bus_Sig/1 -> AC_Compressor_Data_FD1_411/1  "AC_Compressor_Data_FD1_411"
  ElCmprBattSysU_D_Falt/1 -> Bus_Sig/1  "ElCmprBattSysU_D_Falt"
  ElCmprBattURng_D_Falt/1 -> Bus_Sig/2  "ElCmprBattURng_D_Falt"
  ElCmprInnrErr_D_Falt/1 -> Bus_Sig/3  "ElCmprInnrErr_D_Falt"
  ElCmprLostComm_D_Falt/1 -> Bus_Sig/4  "ElCmprLostComm_D_Falt"
  ElCmprOverLoad_D_Falt/1 -> Bus_Sig/5  "ElCmprOverLoad_D_Falt"
  ElCmprOverTe_D_Falt/1 -> Bus_Sig/6  "ElCmprOverTe_D_Falt"
  ElCmprOverTe_D_Stat/1 -> Bus_Sig/7  "ElCmprOverTe_D_Stat"
  ElCmprPerfErr_D_Falt/1 -> Bus_Sig/8  "ElCmprPerfErr_D_Falt"
  ElCmprSysU_D_Falt/1 -> Bus_Sig/9  "ElCmprSysU_D_Falt"
  ElCmprUHi_D_Stat/1 -> Bus_Sig/10  "ElCmprUHi_D_Stat"
  ElCmprUHi_U_Actl/1 -> Bus_Sig/11  "ElCmprUHi_U_Actl"
  ElCmpr_D_Stat/1 -> Bus_Sig/12  "ElCmpr_D_Stat"
  ElCmpr_N_Actl/1 -> Bus_Sig/13  "ElCmpr_N_Actl"
  ElCmpr_Pw_Actl/1 -> Bus_Sig/14  "ElCmpr_Pw_Actl"

== system P702_NI_SoftECU/Input/GWM-SCCM//PDB//RCM//GSM/Other_GWMTx/AC_Compressor_Req_FD1 ==
  Bus_Sig : BusCreator  Inputs=2
  ElCmprEnbl_B_Rq : Constant  Value=0
  ElCmpr_N_Rq : Constant  Value=0
  AC_Compressor_Req_FD1_410 : Outport
  wires:
  Bus_Sig/1 -> AC_Compressor_Req_FD1_410/1  "AC_Compressor_Req_FD1_410"
  ElCmprEnbl_B_Rq/1 -> Bus_Sig/1  "ElCmprEnbl_B_Rq"
  ElCmpr_N_Rq/1 -> Bus_Sig/2  "ElCmpr_N_Rq"

== system P702_NI_SoftECU/Input/GWM-SCCM//PDB//RCM//GSM/Other_GWMTx/APIMGPS_Data_Nav_1_FD1 ==
  Bus_Sig : BusCreator  Inputs=8
  GPS_Latitude_Degrees : Constant  Value=0
  GPS_Latitude_Min_dec : Constant  Value=0
  GPS_Latitude_Minutes : Constant  Value=0
  GPS_Longitude_Degrees : Constant  Value=0
  GPS_Longitude_Min_dec : Constant  Value=0
  GPS_Longitude_Minutes : Constant  Value=0
  GpsHsphLattSth_D_Actl : Constant  Value=0
  GpsHsphLongEast_D_Actl : Constant  Value=0
  APIMGPS_Data_Nav_1_FD1_462 : Outport
  wires:
  Bus_Sig/1 -> APIMGPS_Data_Nav_1_FD1_462/1  "APIMGPS_Data_Nav_1_FD1_462"
  GPS_Latitude_Degrees/1 -> Bus_Sig/1  "GPS_Latitude_Degrees"
  GPS_Latitude_Min_dec/1 -> Bus_Sig/2  "GPS_Latitude_Min_dec"
  GPS_Latitude_Minutes/1 -> Bus_Sig/3  "GPS_Latitude_Minutes"
  GPS_Longitude_Degrees/1 -> Bus_Sig/4  "GPS_Longitude_Degrees"
  GPS_Longitude_Min_dec/1 -> Bus_Sig/5  "GPS_Longitude_Min_dec"
  GPS_Longitude_Minutes/1 -> Bus_Sig/6  "GPS_Longitude_Minutes"
  GpsHsphLattSth_D_Actl/1 -> Bus_Sig/7  "GpsHsphLattSth_D_Actl"
  GpsHsphLongEast_D_Actl/1 -> Bus_Sig/8  "GpsHsphLongEast_D_Actl"

== system P702_NI_SoftECU/Input/GWM-SCCM//PDB//RCM//GSM/Other_GWMTx/APIMGPS_Data_Nav_2_FD1 ==
  Bus_Sig : BusCreator  Inputs=10
  GPS_Actual_vs_Infer_pos : Constant  Value=0
  GPS_Compass_direction : Constant  Value=0
  GPS_Pdop : Constant  Value=0
  GPS_UTC_hours : Constant  Value=0
  GPS_UTC_minutes : Constant  Value=0
  GPS_UTC_seconds : Constant  Value=0
  GpsUtcDay_No_Actl : Constant
  GpsUtcMnth_No_Actl : Constant
  GpsUtcYr_No_Actl : Constant  Value=0
  Gps_B_Falt : Constant  Value=0
  APIMGPS_Data_Nav_2_FD1_463 : Outport
  wires:
  Bus_Sig/1 -> APIMGPS_Data_Nav_2_FD1_463/1  "APIMGPS_Data_Nav_2_FD1_463"
  GPS_Actual_vs_Infer_pos/1 -> Bus_Sig/1  "GPS_Actual_vs_Infer_pos"
  GPS_Compass_direction/1 -> Bus_Sig/2  "GPS_Compass_direction"
  GPS_Pdop/1 -> Bus_Sig/3  "GPS_Pdop"
  GPS_UTC_hours/1 -> Bus_Sig/4  "GPS_UTC_hours"
  GPS_UTC_minutes/1 -> Bus_Sig/5  "GPS_UTC_minutes"
  GPS_UTC_seconds/1 -> Bus_Sig/6  "GPS_UTC_seconds"
  GpsUtcDay_No_Actl/1 -> Bus_Sig/7  "GpsUtcDay_No_Actl"
  GpsUtcMnth_No_Actl/1 -> Bus_Sig/8  "GpsUtcMnth_No_Actl"
  GpsUtcYr_No_Actl/1 -> Bus_Sig/9  "GpsUtcYr_No_Actl"
  Gps_B_Falt/1 -> Bus_Sig/10  "Gps_B_Falt"

== system P702_NI_SoftECU/Input/GWM-SCCM//PDB//RCM//GSM/Other_GWMTx/APIM_Request_Signals_1_FD1 ==
  Bus_Sig : BusCreator  Inputs=6
  ChrgOvrdExitScrn_D_Rq : Constant  Value=0
  EmPrflButtnAssoc_D_Rq : Constant  Value=0
  EmPrflKeyAssoc_D_Rq : Constant  Value=0
  EmPrflNo_D_Rq : Constant  Value=0
  Em_D_Stat : Constant  Value=0
  Rba_D_Rq : Constant  Value=0
  APIM_Request_Signals_1_FD1_227 : Outport
  wires:
  Bus_Sig/1 -> APIM_Request_Signals_1_FD1_227/1  "APIM_Request_Signals_1_FD1_227"
  ChrgOvrdExitScrn_D_Rq/1 -> Bus_Sig/1  "ChrgOvrdExitScrn_D_Rq"
  EmPrflButtnAssoc_D_Rq/1 -> Bus_Sig/2  "EmPrflButtnAssoc_D_Rq"
  EmPrflKeyAssoc_D_Rq/1 -> Bus_Sig/3  "EmPrflKeyAssoc_D_Rq"
  EmPrflNo_D_Rq/1 -> Bus_Sig/4  "EmPrflNo_D_Rq"
  Em_D_Stat/1 -> Bus_Sig/5  "Em_D_Stat"
  Rba_D_Rq/1 -> Bus_Sig/6  "Rba_D_Rq"

== system P702_NI_SoftECU/Input/GWM-SCCM//PDB//RCM//GSM/Other_GWMTx/APIM_Request_Signals_FD1 ==
  Bus_Sig : BusCreator  Inputs=12
  CbnCmrtPrefListIndx_Rq : Constant  Value=0
  CbnCmrtPrefLstNmItm_Rq : Constant  Value=0
  ChargePortPwr_Rq : Constant  Value=0
  ChrgStatDsply_D_Rq : Constant
  FactoryReset_Rq : Constant  Value=0
  LongTermParking_Rq : Constant  Value=0
  ModemReset_D_Rq : Constant  Value=0
  NextUsageTimeToggle_Rq : Constant  Value=0
  OffPeakTimeSetHR_Rq : Constant  Value=0
  OffPeakTimeSetMin_Rq : Constant  Value=0
  StopStrtDrvMde_B_RqBtn3 : Constant  Value=0
  TCU_ESN_D_Rq : Constant  Value=0
  APIM_Request_Signals_FD1_105 : Outport
  wires:
  Bus_Sig/1 -> APIM_Request_Signals_FD1_105/1  "APIM_Request_Signals_FD1_105"
  CbnCmrtPrefListIndx_Rq/1 -> Bus_Sig/1  "CbnCmrtPrefListIndx_Rq"
  CbnCmrtPrefLstNmItm_Rq/1 -> Bus_Sig/2  "CbnCmrtPrefLstNmItm_Rq"
  ChargePortPwr_Rq/1 -> Bus_Sig/3  "ChargePortPwr_Rq"
  ChrgStatDsply_D_Rq/1 -> Bus_Sig/4  "ChrgStatDsply_D_Rq"
  FactoryReset_Rq/1 -> Bus_Sig/5  "FactoryReset_Rq"
  LongTermParking_Rq/1 -> Bus_Sig/6  "LongTermParking_Rq"
  ModemReset_D_Rq/1 -> Bus_Sig/7  "ModemReset_D_Rq"
  NextUsageTimeToggle_Rq/1 -> Bus_Sig/8  "NextUsageTimeToggle_Rq"
  OffPeakTimeSetHR_Rq/1 -> Bus_Sig/9  "OffPeakTimeSetHR_Rq"
  OffPeakTimeSetMin_Rq/1 -> Bus_Sig/10  "OffPeakTimeSetMin_Rq"
  StopStrtDrvMde_B_RqBtn3/1 -> Bus_Sig/11  "StopStrtDrvMde_B_RqBtn3"
  TCU_ESN_D_Rq/1 -> Bus_Sig/12  "TCU_ESN_D_Rq"

== system P702_NI_SoftECU/Input/GWM-SCCM//PDB//RCM//GSM/Other_GWMTx/APIM_Send_Signals1_FD1 ==
  APIM_ActiveTrackNum_St : Constant  Value=0
  APIM_NumberofTracks_St : Constant  Value=0
  AutoHoldSwtch_D_Stat3 : Constant  Value=0
  Bus_Sig : BusCreator  Inputs=9
  CenterStackRing_D_Actl : Constant  Value=2
  ChrgCordUnlock_B_Rq : Constant  Value=0
  TrlrAidCancl_B_Rq : Constant  Value=0
  TrlrAidSetup_D_Stat : Constant  Value=0
  TrlrTrgtAcquire_D_Rq : Constant  Value=0
  ValetMode_D_Stat : Constant  Value=0
  APIM_Send_Signals1_FD1_3F1 : Outport
  wires:
  Bus_Sig/1 -> APIM_Send_Signals1_FD1_3F1/1  "APIM_Send_Signals1_FD1_3F1"
  APIM_ActiveTrackNum_St/1 -> Bus_Sig/1  "APIM_ActiveTrackNum_St"
  APIM_NumberofTracks_St/1 -> Bus_Sig/2  "APIM_NumberofTracks_St"
  AutoHoldSwtch_D_Stat3/1 -> Bus_Sig/3  "AutoHoldSwtch_D_Stat3"
  CenterStackRing_D_Actl/1 -> Bus_Sig/4  "CenterStackRing_D_Actl"
  ChrgCordUnlock_B_Rq/1 -> Bus_Sig/5  "ChrgCordUnlock_B_Rq"
  TrlrAidCancl_B_Rq/1 -> Bus_Sig/6  "TrlrAidCancl_B_Rq"
  TrlrAidSetup_D_Stat/1 -> Bus_Sig/7  "TrlrAidSetup_D_Stat"
  TrlrTrgtAcquire_D_Rq/1 -> Bus_Sig/8  "TrlrTrgtAcquire_D_Rq"
  ValetMode_D_Stat/1 -> Bus_Sig/9  "ValetMode_D_Stat"

== system P702_NI_SoftECU/Input/GWM-SCCM//PDB//RCM//GSM/Other_GWMTx/APIM_Send_Signals_2_FD1 ==
  Bus_Sig : BusCreator  Inputs=15
  OnbChrgClearAll_B_Rq : Constant  Value=0
  OnbChrgGoTDelete_B_Rq : Constant  Value=0
  OnbChrgGoTElement_D_Rq : Constant  Value=0
  OnbChrgGoTExtHtr_D_Rq : Constant  Value=0
  OnbChrgGoTHr_T_Rq : Constant  Value=30
  OnbChrgGoTMnte_D_Rq : Constant  Value=0
  OnbChrgGoTOn_D_Rq : Constant  Value=2
  OnbChrgGoTPrcond_D_Rq : Constant  Value=0
  OnbChrgGoTTouch_D_Rq : Constant  Value=0
  OnbChrgGoTUpdate_B_Rq : Constant  Value=0
  OtaTrg_D_Stat : Constant  Value=0
  PaakMyKey_D_Rq : Constant  Value=0
  TCU_Final_Actvtn_St : Constant  Value=0
  TCU_Init_Actvtn_St : Constant  Value=0
  TrlrAidMde_D_Rq : Constant  Value=0
  APIM_Send_Signals_2_FD1_215 : Outport
  wires:
  Bus_Sig/1 -> APIM_Send_Signals_2_FD1_215/1  "APIM_Send_Signals_2_FD1_215"
  OnbChrgClearAll_B_Rq/1 -> Bus_Sig/1  "OnbChrgClearAll_B_Rq"
  OnbChrgGoTDelete_B_Rq/1 -> Bus_Sig/2  "OnbChrgGoTDelete_B_Rq"
  OnbChrgGoTElement_D_Rq/1 -> Bus_Sig/3  "OnbChrgGoTElement_D_Rq"
  OnbChrgGoTExtHtr_D_Rq/1 -> Bus_Sig/4  "OnbChrgGoTExtHtr_D_Rq"
  OnbChrgGoTHr_T_Rq/1 -> Bus_Sig/5  "OnbChrgGoTHr_T_Rq"
  OnbChrgGoTMnte_D_Rq/1 -> Bus_Sig/6  "OnbChrgGoTMnte_D_Rq"
  OnbChrgGoTOn_D_Rq/1 -> Bus_Sig/7  "OnbChrgGoTOn_D_Rq"
  OnbChrgGoTPrcond_D_Rq/1 -> Bus_Sig/8  "OnbChrgGoTPrcond_D_Rq"
  OnbChrgGoTTouch_D_Rq/1 -> Bus_Sig/9  "OnbChrgGoTTouch_D_Rq"
  OnbChrgGoTUpdate_B_Rq/1 -> Bus_Sig/10  "OnbChrgGoTUpdate_B_Rq"
  OtaTrg_D_Stat/1 -> Bus_Sig/11  "OtaTrg_D_Stat"
  PaakMyKey_D_Rq/1 -> Bus_Sig/12  "PaakMyKey_D_Rq"
  TCU_Final_Actvtn_St/1 -> Bus_Sig/13  "TCU_Final_Actvtn_St"
  TCU_Init_Actvtn_St/1 -> Bus_Sig/14  "TCU_Init_Actvtn_St"
  TrlrAidMde_D_Rq/1 -> Bus_Sig/15  "TrlrAidMde_D_Rq"

== system P702_NI_SoftECU/Input/GWM-SCCM//PDB//RCM//GSM/Other_GWMTx/ActiveFrontStrg_Stat2_FD1 ==
  Bus_Sig : BusCreator  Inputs=2
  SteWhlRelCalib_An_Sns : Constant  Value=0
  SteWhlRelCalib_T_Actl : Constant  Value=0
  ActiveFrontStrg_Stat2_FD1_8A : Outport
  wires:
  Bus_Sig/1 -> ActiveFrontStrg_Stat2_FD1_8A/1  "ActiveFrontStrg_Stat2_FD1_8A"
  SteWhlRelCalib_An_Sns/1 -> Bus_Sig/1  "SteWhlRelCalib_An_Sns"
  SteWhlRelCalib_T_Actl/1 -> Bus_Sig/2  "SteWhlRelCalib_T_Actl"
